simulink model "Ex1s"  (R2025a)
settings: Solver=VariableStepAuto  StartTime=0.0  StopTime=10.0  RelTol=1e-3
values from neighbouring files (symbols this model uses):
  sys1 = linearize('Ex1s',io1,op1)    [Ex1.m]

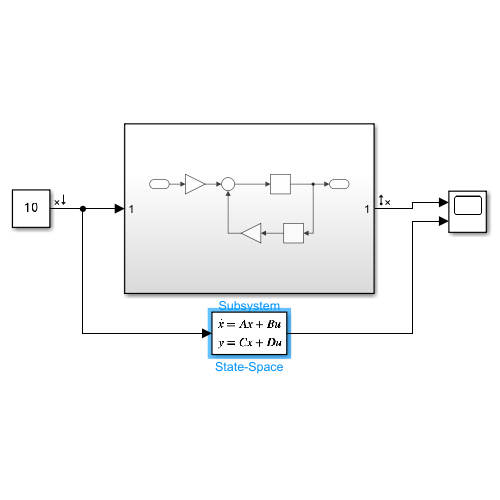
[thumbnail: Simulink's stored preview of the top-level diagram]
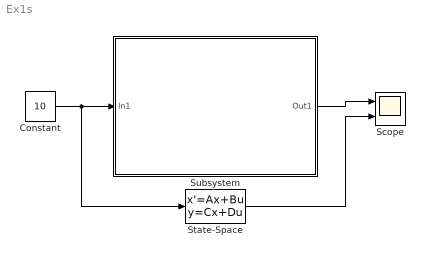
== system Ex1s ==
  Constant : Constant  Value=10
  Scope : Scope  NumInputPorts=2
      settings: ActiveDisplayYMinimum=0.35225922520471742  ActiveDisplayYMaximum=6.8296669731575452
  State-Space : StateSpace  A=sys1.A  B=sys1.B  C=sys1.C  D=sys1.D  InitialCondition=1
  Subsystem : Subsystem
  wires:
  Subsystem/1(Out1) -> Scope/1
  Constant/1 -> State-Space/1, Subsystem/1(In1)
  State-Space/1 -> Scope/2

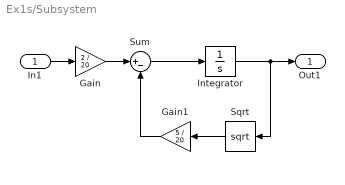
== system Ex1s/Subsystem ==
  In1 : Inport
  Gain : Gain  Gain=2 / 20
  Gain1 : Gain  Gain=5 / 20
  Integrator : Integrator  InitialCondition=1
  Sqrt : Sqrt
  Sum : Sum  Inputs=|+-
  Out1 : Outport
  wires:
  In1/1 -> Gain/1
  Gain/1 -> Sum/1
  Sum/1 -> Integrator/1
  Integrator/1 -> Sqrt/1, Out1/1
  Sqrt/1 -> Gain1/1
  Gain1/1 -> Sum/2
